simulink model "StateEstimationFilter"  (R2019b)
settings: Solver=VariableStepAuto  StartTime=0.0  StopTime=117  FixedStep=0.001  RelTol=1e-3
PostLoadFcn:
  | , if any(exist('dsrtsu_mdlpostloadfcn', 'file') == [2, 3, 6]), try dsrtsu_mdlpostloadfcn('Execute', bdroot); catch fprintf('Error in PostLoadFcn (dsrtsu_mdlpostloadfcn) for model "%s":\n %s\n', bdroot, lasterr); end, end,
InitFcn:
  | , if any(exist('rtifpga_mdlclblib', 'file') ~= 0), rtifpga_mdlclblib('Init', bdroot); end,
Description:
  | Standard RTI1401 template.
  | Supported MATLAB version:  R2020a.
settings Model: Tag=RTI1401  DSRTSU_INTERNAL_RTI_VER=580  DSRTSU_INTERNAL_RTI_TYPE=rti1401  RTICANMMDATA=struct('GeneralSetupData',struct('modelroot','C:\Users\soso7\Desktop','generalsettings',struct('filesettings',struct('destfolder',struct('Name','RTICANMM_FILES','Check',1),'buildfolder',struct('Name','.','Check',1),'AbsDestfolder',struct('Name','C:\Users\soso7\Desktop\RTICANMM_FILES'),'AbsBuildfolder',struct('Name','C:\Users\soso7\Desktop'))),'options',struct('addpaths',1,'rmpaths',1,'addtrcexclusion',true,'cannavigator',struct('checkmonitoring',0),'show_usrtrc',0,'use_usrtrc',0),'advanced',struct('options',ones(1,100)),'MPSetup',{{}},'RTI',struct('Type','RTI1401','Ver','7.16','Date','02-May-2021'),'modelname','Kalman','block','Kalman'))  DSRTSU_INTERNAL_RTIFPGA=170  Creator=soso7  LastModifiedBy=cosimulation
settings DataIOCC: ReturnWorkspaceOutputs=off
settings OptimizationCC: BlockReduction=off  OptimizeBlockIOStorage=off  BufferReuse=off  GlobalBufferReuse=off  ExpressionFolding=off  LocalBlockOutputs=off  OptimizeDataStoreBuffers=off  BusAssignmentInplaceUpdate=off
settings DebuggingCC: ArithmeticOperatorsInVariantConditions=warning
settings HardwareCC: ProdBitPerPointer=32  ProdBitPerSizeT=32  ProdBitPerPtrDiffT=32  ProdLargestAtomicInteger=Integer  ProdEndianess=BigEndian  ProdWordSize=32  ProdLongLongMode=on  ProdHWDeviceType=Custom Processor->Custom  TargetIntDivRoundTo=Zero  TargetEndianess=BigEndian  TargetHWDeviceType=Custom Processor->Custom
settings ModelReferenceCC: EnableParallelModelReferenceBuilds=on  ParallelModelReferenceMATLABWorkerInit=Load Top Model
settings SFSimCC: SimUseLocalCustomCode=off  MATLABDynamicMemAlloc=off  CustomCodeUndefinedFunction=UseInterfaceOnly
settings RTWCC: Description=dSPACE DS1401 Hardware Platform  SystemTargetFile=rti1401.tlc  MakeCommand=make_rti  TemplateMakefile=rti1401.tmf  RTWUseLocalCustomCode=off
settings CodeAppCC: StateflowObjectComments=on
settings STFCustomTargetCC: ParMdlRefBuildCompliant=on  SystemTargetFile=rti1401.tlc
settings GRTTargetCC: TargetLangStandard=C89/C90 (ANSI)  CompOptLevelCompliant=off  ConcurrentExecutionCompliant=off  CombineOutputUpdateFcns=off  MatFileLogging=off  CPPClassGenCompliant=off  UseToolchainInfoCompliant=off
settings ConfigComp: CovMetricSettings=dswe

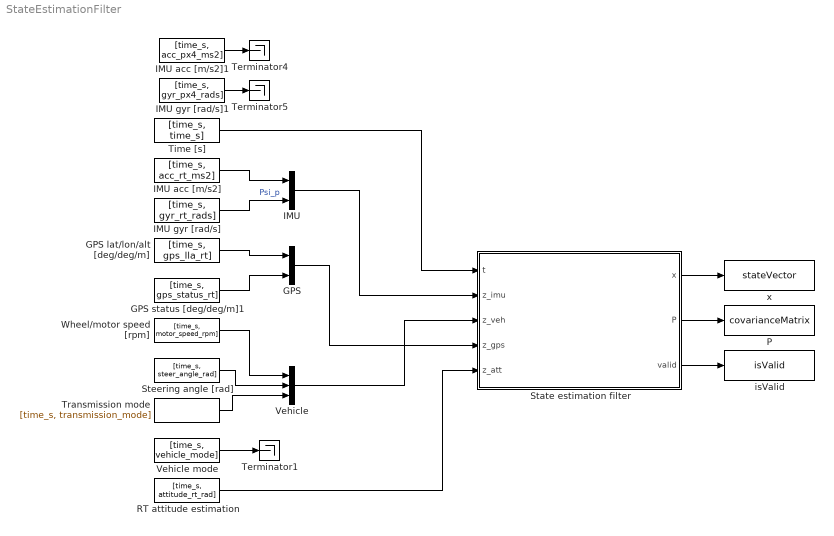
== system StateEstimationFilter ==
  GPS : Concatenate
  GPS lat/lon/alt [deg/deg/m] : FromWorkspace  VariableName=[time_s, gps_lla_rt]  SampleTime=0
  GPS status [deg/deg/m]1 : FromWorkspace  VariableName=[time_s, gps_status_rt]  SampleTime=0
  IMU : Concatenate
  IMU acc [m/s2] : FromWorkspace  VariableName=[time_s, acc_rt_ms2]  SampleTime=0
  IMU acc [m/s2]1 : FromWorkspace  VariableName=[time_s, acc_px4_ms2]  SampleTime=0
  IMU gyr [rad/s] : FromWorkspace  VariableName=[time_s, gyr_rt_rads]  SampleTime=0
  IMU gyr [rad/s]1 : FromWorkspace  VariableName=[time_s, gyr_px4_rads]  SampleTime=0
  P : ToWorkspace  VariableName=covarianceMatrix  SaveFormat=Timeseries  SampleTime=-1
  RT attitude estimation : FromWorkspace  VariableName=[time_s, attitude_rt_rad]  SampleTime=0
  State estimation filter : MATLAB Function  TreatAsAtomicUnit=on  SystemSampleTime=0.01
  Steering angle [rad] : FromWorkspace  VariableName=[time_s, steer_angle_rad]  SampleTime=0
  Terminator1 : Terminator
  Terminator4 : Terminator
  Terminator5 : Terminator
  Time [s] : FromWorkspace  VariableName=[time_s, time_s]  SampleTime=0
  Transmission mode : FromWorkspace  VariableName=[time_s, transmission_mode]  SampleTime=0
  Vehicle : Concatenate  NumInputs=3
  Vehicle mode : FromWorkspace  VariableName=[time_s, vehicle_mode]  SampleTime=0
  Wheel/motor speed [rpm] : FromWorkspace  VariableName=[time_s, motor_speed_rpm]  SampleTime=0
  isValid : ToWorkspace  VariableName=isValid  SaveFormat=Timeseries  SampleTime=-1
  x : ToWorkspace  VariableName=stateVector  SaveFormat=Timeseries  SampleTime=-1
  wires:
  Time [s]/1 -> State estimation filter/1(t)
  IMU acc [m/s2]1/1 -> Terminator4/1
  IMU gyr [rad/s]1/1 -> Terminator5/1
  IMU acc [m/s2]/1 -> IMU/1
  IMU gyr [rad/s]/1 -> IMU/2  "Psi_p"
  IMU/1 -> State estimation filter/2(z_imu)
  GPS lat/lon/alt [deg/deg/m]/1 -> GPS/1
  GPS status [deg/deg/m]1/1 -> GPS/2
  GPS/1 -> State estimation filter/4(z_gps)
  Wheel/motor speed [rpm]/1 -> Vehicle/1
  Steering angle [rad]/1 -> Vehicle/2
  Transmission mode/1 -> Vehicle/3
  Vehicle/1 -> State estimation filter/3(z_veh)
  State estimation filter/1(x) -> x/1
  State estimation filter/2(P) -> P/1
  State estimation filter/3(valid) -> isValid/1
  Vehicle mode/1 -> Terminator1/1
  RT attitude estimation/1 -> State estimation filter/5(z_att)

== matlab function StateEstimationFilter/State estimation filter ==
  data: x output; P output; t input; z_imu input; z_veh input; z_gps input; valid output; z_att input
function [x, P, valid] = stateEstimationFilterFunc(t, z_imu, z_veh, z_gps, z_att)
[x, P, valid] = stateEstimationFilter(t, z_imu, z_veh, z_gps, z_att);
end
